simulink library "commsource"  (Simulink 5.0)
values from neighbouring files (symbols this model uses):
  m1 = sqrt(2*K(:)).*s    [commblkriciansrc.m]
  m2 = 0    [commblkriciansrc.m]
  ts = td(1)    [commblkreadwkspc.m]    (also in eyediasi.m = [-1, 0]; eyesampl.m = [sampleTime(1), sampleTime(2)])
undefined symbols (not defined in the file or in its folder): randint
libraries: commsource x4, dspsrcs2 x3, commutil x1, dspbdsp2 x1
settings Model: Creator=tdelve  LastModifiedBy=mmclerno

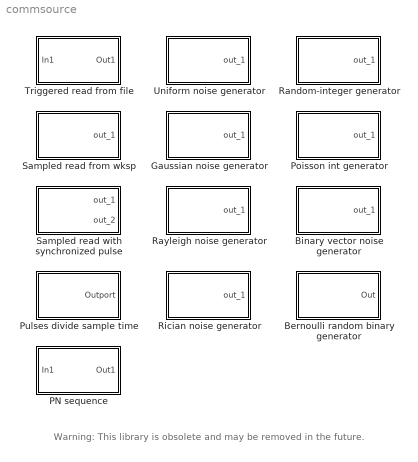
== system commsource ==
  note: Warning:  This library is obsolete and may be
      | removed in the future.
  Bernoulli random binary generator : Subsystem  mask(Bernoulli binary random number generator){P=[0.1 0.5], Seed=[1 2], Ts=1}
      mask prompts: P "Probability of a zero:"; Ts "Sample time (s):"
      mask help:
      | Generate a Bernoulli random binary number.
      | To generate a vector output, specify the probability as a vector.
      mask init:
      | [L,U,Seed,x,y]=commblkbernoullisrc(gcb,'init',{P,Seed});
      mask Help: The Bernoulli binary random number generator outputs random binary numbers. The first parameter is the probability of a zero. This parameter can be specified as a vector to produce an output vector of the same size. The seed can be either a scalar or a vector of the same size as the probability vector.
      mask Display: plot(0,0,100,100,x,y);disp('Bernoulli bin')
  Binary vector noise generator : Subsystem  mask(Binary noise generator){n=7, prob=0.5, seed=12345, Ts=1}
      mask prompts: n "Binary vector length:"; prob "Probability of a "one", two "ones",three "ones"...:"; Ts "Sample time (s):"
      mask help: Generate a binary vector with control over the number of "1"s.
      mask init:
      | [x,y]=commblkrandbitsrc(gcb,'init');
      mask Help: This block outputs a zero vector with "1"s randomly distributed the vector. The maximum number of "1"s in the vector is the same as the length of the vector probability. The value of the ith element of the probability is the probability of i number of "1"s in the vector, e.g. [1/4 1/4 1/4] means probability of single "1", double "1"s, three "1"s or no "1" in the vector is 1/4.
      mask Display: plot(0,0,100,100,x,y);disp('B-vector')
  Gaussian noise generator : Subsystem  mask(Gaussian noise generator){m=[0 1], d=[1 2], s=[100 200], Ts=1}
      mask prompts: m "Mean value:"; d "Variance (vector or matrix):"; s "Initial seed:"; Ts "Sample time (s):"
      mask help: Generate Gaussian distributed noise with given mean and variance value.
      mask init:
      | [m,d,s]=commblkgaussiansrc(gcb,'init',{m,d,s});
      mask Help: When the mean value and seed are vectors, the output of this block is a vector. The length of the vector is the same as the length of the mean value vector or the length of the seed. When the variance entry is a vector, the variance is a diagonal matrix.
      mask Display:
      | plot(0,0,100,100,[95 5 10 10 10 (100-15)*[0:1/30:1]+10],[75 75 75 70 95 randn(1,31)*10+75]);
      | disp('\nGaussian')
  PN sequence : Subsystem  mask(Pseudorandom sequence generator){M=2, poly=[0 -5 -6], ini_sta=[1 1 0 1 0 1]}
      mask prompts: M "Calculation base:"; poly "Generator polynomial:"; ini_sta "Initial states"
      mask help: This block outputs a sequence of pseudorandom symbols. The rising edge of the input synchronization pulse triggers the register shifting in the block to update the output.
      mask init:
      | if M<=0, error('Scramble calculation base must be a positive integer.'); end
      | if max(poly)>=M
      |  error('Scramble polynomial coefficients must be less than calculation base.');
      | elseif min(poly)<0
      |   tmp = zeros(1, abs(min(poly))+1);
      |   for i = 1:length(poly), tmp(abs(poly(i))+1) = 1; end
      |   poly = tmp;
      | end
      | if poly(1) == 0, poly(1) = 1; end
      | s = length(poly)-1;
      mask Help: A pseudorandom sequence can be used for a direct sequence spread spectrum system. Its operation is based on a generator polynomial g(x).  You can specify the polynomial using the coefficients of the polynomial or by specifying the terms for which the coefficient is 1; for other terms, the coefficient is the default, 0. For example g = [1 0 0 0 0 0 1 0 1] and g = [0 -6 -8] represent the same polynomial g(x) = 1 + x^(-6) + x^(-8). The initial state of at least one of the registers must be nonzero in order to generate a nonzero sequence.
      mask Display:
      | disp('Pseudorandom\nsequence\ngenerator')
      | plot(0,0,100,100,[5 10 10 8 10 12 10 10 15]-5,[5 5 12 8 12 8 12 15 15]+40)
  Poisson int generator : Subsystem  mask(Poisson random integer generator){lambda=[0.1 3], seed=[1 2], Ts=1}
      mask prompts: Ts "Sample time (s):"
      mask help: Generate Poisson distributed random integers.
      mask init:
      | [x,y]=commblkpoissonsrc(gcb,'init');
      mask Help: This block generates Poisson distributed integer values. The output size is the same as the seed vector size. The variance and mean value equal to Lambda. Add a limiter to the output of this block to generate binary noise.
      mask Display: plot(0,0,100,100,x,y);disp('Poisson int')
  Pulses divide sample time : Subsystem  mask(Pulse generator){samp_time=1, out_divid=[1 3 5 1 3 5], offset=[0 0 0 4.1 2.1 4.1]}
      mask prompts: samp_time "Sample time (scalar, sec):"; out_divid "Divider (integer vector):"; offset "Offset (same length as Divider):"
      mask help:
      | Vector pulses with sample rate of each pulse as
      | Sample_time / Divider.
      mask init:
      | [x,y]=srcsicon(2);
      mask Help: This block generates a vector pulse. The output length is the same as the divider vector length. The ith element of the output has the sample time Sample_time/Divider(i). All elements in divider must be integers.
      mask Display: plot(0,0,100,100,x,y);disp('Pulse')
  Random-integer generator : Subsystem  mask(Random integer generator){mul=8, seed=[1 2], Ts=1}
      mask prompts: mul "M-ary number:"; Ts "Sample time (s):"
      mask help: Generate integers randomly distributed in range [0, M-1], where M is the M-ary number.
      mask init:
      | [x,y]=commblkrandintsrc(gcb,'init');
      mask Help: This block generates an integer number in the range [0 M-1], where M is the M-ary number. The probability of the appearance for each number is equal.
      mask Display: plot(0,0,100,100,x,y);disp('Random int')
  Rayleigh noise generator : Subsystem  mask(Rayleigh noise generator){alpha=1, seed=17658, Ts=1}
      mask prompts: alpha "sigma:"; seed "Initial seed:"; Ts "Sample time (s):"
      mask help: Generate Rayleigh distributed noise.The output vector size of this block is the same as the vector size of the seed.
      mask init:
      | [alpha,seed]=commblkrayleighsrc(gcb,'init',{alpha,seed});
      mask Help: This block generates Rayleigh noise with the given sigma value. The sigma value is the standard deviations of the zero mean Gaussian noise components in generating the Rayleigh noise. The output vector size of this block is the same as the vector size of the seed.
      mask Display: plot(0,0,100,100,[95 5 10 10 10 (100-15)*[0:1/30:1]+10],[75 75 75 70 95 rand(1,31)*20+75]);disp('Rayleigh')
  Rician noise generator : Subsystem  mask(Rician noise generator){specMethod=K-factor, iMean=sqrt(2), qMean=sqrt(2), K=2, s=1, seed=12345, Ts=1}
      mask prompts: specMethod "Specification method:"; iMean "In phase component (mean):"; qMean "Quadrature component (mean):"; K "Rician K-factor:"; s "sigma:"; Ts "Sample time (s):"
      mask help: Generate Rician distributed noise. The output vector size of this block is the same as the vector size of the seed.
      mask init:
      | [m1, m2]=commblkriciansrc(gcb,'init',{iMean, qMean, K, s});
      mask Help:
      | The Rician noise is composed with two independant Gaussian noises. These two Gaussain noises have a same std, sigma. Their mean values are m1 and m2 respectively.
      | 
      | Where where Rician K-factor is used, K-Factor=(m1^2+m2^2)/2/sigma^2.
      | 
      | The output vector size of this block is the same as the vector size of the seed.
      mask StyleString: popup(K-factor|Quadrature components),edit,edit,edit,edit,edit,edit
      mask CallbackString: commblkriciansrc(gcb,'SpecMethod');||||||
      mask Display:
      | plot(0,0,100,100,[95 5 10 10 10 (100-15)*[0:1/30:1]+10],[75 75 75 70 95 rand(1,31)*20+75]);
      | disp('Rician');
  Sampled read from wksp : Subsystem  mask(Sampled read from workspace){X=randint(1000,1,2), td=1, cyc=off}
      mask prompts: X "Signal:"; td "Data output sample time (sec):"; cyc "Cyclic repeat"
      mask help: Read from a workspace variable at a specified sampling interval.
      mask init:
      | commblkreadwkspc;
      mask Help: This block reads from a workspace variable at a given sample time. If the workspace variable is a matrix, the size of the block output vector corresponds to the number of columns in the matrix. If the "Cyclic repeat" box is checked, after reading the last row of the variable the block will  return to the first row of the variable.  Otherwise, the block will output zeros after reading the last row of the variable.
      mask Display: plot(0,0,100,100,[5+[20 20 0 0 2 7 2 7 2 7 12 7 12 7 20 20],[0:1/30:1]*70+25],[10 20 20 0 0 9 16 9 0 0 9 16 9 0 0 8,sin(6.28*[0:1/30:1])*10+10]+65);disp('\nRd wksp')
  Sampled read with synchronized pulse : Subsystem  mask(Sampled read from workspace with synchronized pulse){X=randint(300,1,2), td=1, cyc=off}
      mask prompts: X "Signal:"; td "Data output sample time (sec):"; cyc "Cyclic repeat"
      mask help: Read from a workspace variable at a specified sampling interval.
      mask init:
      | [x,y]=trigicon(1,75,get_param(gcb,'orientation'),2);
      | commblkreadwkspc;
      mask Help: This block reads from a workspace variable at a given sample time. If the workspace variable is a matrix, the size of the block output vector corresponds to the number of columns in the matrix. If the "Cyclic repeat" box is checked, after reading the last row of the variable the block will  return to the first row of the variable.  Otherwise, the block will output zeros after reading the last row of the variable.  The second output is the synchronization pulse, which provides a rising edge coincident with the data.
      mask Display: plot(0,0,100,100,[5+[20 20 0 0 2 7 2 7 2 7 12 7 12 7 20 20],[0:1/30:1]*70+25],[10 20 20 0 0 9 16 9 0 0 9 16 9 0 0 8,sin(6.28*[0:1/30:1])*10+10]+65,x,y); disp('\nRd wksp')
  Triggered read from file : Subsystem  mask(Read from file){filename='junk.tmp', datatype='ascii', dec=1, numout=1, recursive=off, threshold=.3}
      mask prompts: filename "File name (string, include extension):"; datatype "Data type ('ascii','float','integer'):"; dec "Decimation:"; numout "Output vector length:"; recursive "Cyclic repeat"; threshold "Threshold in detecting trigger signal:"
      mask help: The rising edge of the signal from the 2nd port triggers the block to read the next row of the specified file.
      mask init:
      | [x,y]=trigicon(0,50,get_param(gcb,'orientation'),2);
      | nump = dec - 1;
      mask Help: This block reads the data from a file. The output is refreshed at the rising edge of the input pulse. When the end of the file (eof) is reached, you can have the block output all zeros or start from the beginning of the file.
      mask Display:
      | plot(0,0,100,100,[25 25 05 05 25 25 05 13 13 17 17 17 15 real(exp(j*pi*([0:20]/10+1/2)))*3.5+15 15 25 25 25+[0:1/30:1]*70], [85 95 95 75 75 89 89 89 95 95 89 89 89 imag(exp(j*pi*([0:20]/10+1/2)))*3.5+85 89 89 85 sin([0:1/30:1]*pi*2)*10+85]-10,x,y);
      | disp(' \nRd file')
  Uniform noise generator : Subsystem  mask(Uniform noise generator){low=[0 1], up=[1 2], seed=[12345 54321], Ts=1}
      mask prompts: low "Noise lower bound:"; up "Noise upper bound:"; Ts "Sample time (s):"
      mask help: Generate uniformly distributed noise between the upper and lower bounds.
      mask init:
      | commblkuniformsrc(gcb,'init');
      mask Help: This block generates a uniformly distributed noise between the given lower and upper bounds. The output size is the same as the vector length of the seed. The upper bound and lower bound can be scalar or vectors with their lengths the same as the length for the seed. The vector length of upper bound must be the same as length of lower bound.
      mask Display: plot(0,0,100,100,[95 5 10 10 10 (100-15)*[0:1/30:1]+10],[75 75 75 70 95 rand(1,31)*20+75]);disp('Uniform')

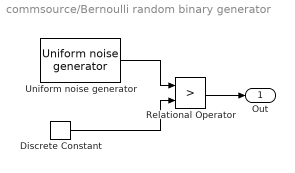
== system commsource/Bernoulli random binary generator ==
  Discrete Constant : dspsrcs2/Discrete Constant  Value=P  Ts=Ts
  Relational Operator : RelationalOperator  Operator=>  InputSameDT=on
  Uniform noise generator : commsource/Uniform noise generator  low=L  up=U  seed=Seed  Ts=Ts
  Out : Outport
  wires:
  Uniform noise generator/1 -> Relational Operator/1
  Discrete Constant/1 -> Relational Operator/2
  Relational Operator/1 -> Out/1

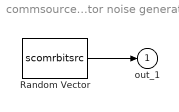
== system commsource/Binary vector noise generator ==
  Random Vector : S-Function  FunctionName=scomrbitsrc  Parameters=n, prob, seed,Ts
  out_1 : Outport  InitialOutput=0
  wires:
  Random Vector/1 -> out_1/1

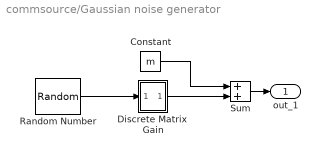
== system commsource/Gaussian noise generator ==
  Constant : Constant  Value=m
  Discrete Matrix  Gain : Subsystem  mask(Discrete Matrix Gain){K=d, Ts=Ts}
      mask prompts: K "Gain Matrix:"; Ts "Sample time (s):"
      mask Display: disp('K')
  Random Number : RandomNumber  Seed=s  SampleTime=Ts
  Sum : Sum  SaturateOnIntegerOverflow=on  InputSameDT=on
  out_1 : Outport  InitialOutput=0
  wires:
  Constant/1 -> Sum/1
  Random Number/1 -> Discrete Matrix  Gain/1(In)
  Discrete Matrix  Gain/1(Out) -> Sum/2
  Sum/1 -> out_1/1

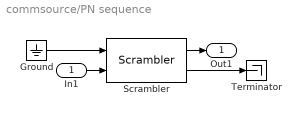
== system commsource/PN sequence ==
  In1 : Inport
  Ground : Ground
  Scrambler : commutil/Scrambler  M=M  poly=poly  ini_sta=ini_sta
  Terminator : Terminator
  Out1 : Outport  InitialOutput=0
  wires:
  In1/1 -> Scrambler/2
  Scrambler/1 -> Out1/1
  Scrambler/2 -> Terminator/1
  Ground/1 -> Scrambler/1

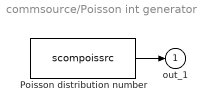
== system commsource/Poisson int generator ==
  Poisson distribution number : S-Function  FunctionName=scompoissrc  Parameters=seed,lambda,Ts
  out_1 : Outport  InitialOutput=0
  wires:
  Poisson distribution number/1 -> out_1/1

== system commsource/Pulses divide sample time ==
  S-function1 : S-Function  FunctionName=homopuls  Parameters=samp_time, out_divid, offset
  Outport : Outport  InitialOutput=0
  wires:
  S-function1/1 -> Outport/1

== system commsource/Random-integer generator ==
  Uniform number : S-Function  FunctionName=scomrintsrc  Parameters=seed,mul,Ts
  out_1 : Outport  InitialOutput=0
  wires:
  Uniform number/1 -> out_1/1

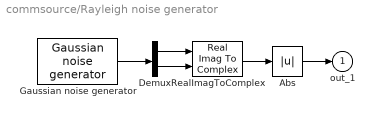
== system commsource/Rayleigh noise generator ==
  Abs : Abs  SaturateOnIntegerOverflow=on
  Demux : Demux  Outputs=2
  Gaussian noise generator : commsource/Gaussian noise generator  m=0  d=alpha  s=seed  Ts=Ts
  RealImagToComplex : RealImagToComplex
  out_1 : Outport  InitialOutput=0
  wires:
  RealImagToComplex/1 -> Abs/1
  Abs/1 -> out_1/1
  Gaussian noise generator/1 -> Demux/1
  Demux/1 -> RealImagToComplex/1
  Demux/2 -> RealImagToComplex/2

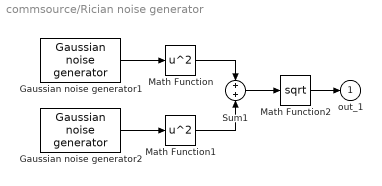
== system commsource/Rician noise generator ==
  Gaussian noise generator1 : commsource/Gaussian noise generator  m=m1  d=s  s=seed  Ts=Ts
  Gaussian noise generator2 : commsource/Gaussian noise generator  m=m2  d=s  s=seed+max(seed)  Ts=Ts
  Math Function : Math  Operator=square
  Math Function1 : Math  Operator=square
  Math Function2 : Math  Operator=sqrt
  Sum1 : Sum  SaturateOnIntegerOverflow=on  InputSameDT=on
  out_1 : Outport  InitialOutput=0
  wires:
  Gaussian noise generator1/1 -> Math Function/1
  Gaussian noise generator2/1 -> Math Function1/1
  Sum1/1 -> Math Function2/1
  Math Function/1 -> Sum1/1
  Math Function1/1 -> Sum1/2
  Math Function2/1 -> out_1/1

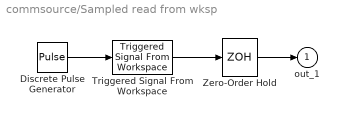
== system commsource/Sampled read from wksp ==
  Discrete Pulse Generator : DiscretePulseGenerator  SampleTime=ts
  Triggered Signal From Workspace : dspsrcs2/Triggered Signal From Workspace  X=X  trigtype=Either edge  cyclic=off  ic=ic  nsamps=SamplesPerFrame
  Zero-Order Hold : ZeroOrderHold  SampleTime=[ts off]
  out_1 : Outport  InitialOutput=0
  wires:
  Zero-Order Hold/1 -> out_1/1
  Triggered Signal From Workspace/1 -> Zero-Order Hold/1
  Discrete Pulse Generator/1 -> Triggered Signal From Workspace/1

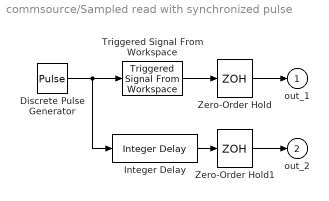
== system commsource/Sampled read with synchronized pulse ==
  Discrete Pulse Generator : DiscretePulseGenerator  SampleTime=ts/2
  Integer Delay : dspbdsp2/Integer Delay  delay=off>(ts/2)  ic=0  frame=off  df=on  numChans=1
  Triggered Signal From Workspace : dspsrcs2/Triggered Signal From Workspace  X=X  trigtype=Rising edge  cyclic=off  ic=ic  nsamps=SamplesPerFrame
  Zero-Order Hold : ZeroOrderHold  SampleTime=[ts off]
  Zero-Order Hold1 : ZeroOrderHold  SampleTime=[ts/2 rem(off,ts/2)]
  out_1 : Outport  InitialOutput=0
  out_2 : Outport  Port=2  InitialOutput=0
  wires:
  Zero-Order Hold1/1 -> out_2/1
  Discrete Pulse Generator/1 -> Triggered Signal From Workspace/1, Integer Delay/1
  Triggered Signal From Workspace/1 -> Zero-Order Hold/1
  Zero-Order Hold/1 -> out_1/1
  Integer Delay/1 -> Zero-Order Hold1/1

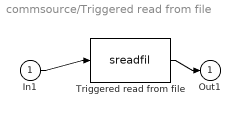
== system commsource/Triggered read from file ==
  In1 : Inport
  Triggered read from file : S-Function  FunctionName=sreadfil  Parameters=filename,datatype,nump,numout,recursive,threshold
  Out1 : Outport  InitialOutput=0
  wires:
  In1/1 -> Triggered read from file/1
  Triggered read from file/1 -> Out1/1

== system commsource/Uniform noise generator ==
  Uniform noise : S-Function  FunctionName=scomunisrc  Parameters=seed,up,low,Ts
  out_1 : Outport  InitialOutput=0
  wires:
  Uniform noise/1 -> out_1/1

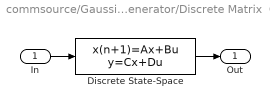
== system commsource/Gaussian noise generator/Discrete Matrix  Gain ==
  In : Inport
  Discrete State-Space : DiscreteStateSpace  A=[]  B=[]  C=[]  D=K  SampleTime=Ts
  Out : Outport
  wires:
  Discrete State-Space/1 -> Out/1
  In/1 -> Discrete State-Space/1
